simulink model "virtual_nonVirtual_CodeGeneration"  (R2024a)
settings: Solver=FixedStepDiscrete  StartTime=0.0  StopTime=10.0  FixedStep=0.5  MaxStep=1  RelTol=1
settings Model: Creator=DELL  LastModifiedBy=DELL
settings OptimizationCC: DefaultParameterBehavior=Inlined  EnhancedBackFolding=on  PassReuseOutputArgsAs=Individual arguments  ZeroExternalMemoryAtStartup=off  ZeroInternalMemoryAtStartup=off  OptimizeBlockOrder=speed  DifferentSizesBufferReuse=on  OptimizationCustomize=off  EfficientTunableParamExpr=on
settings DebuggingCC: ParameterTunabilityLossMsg=error
settings SFSimCC: MATLABDynamicMemAlloc=off
settings RTWCC: Description=Embedded Coder  SystemTargetFile=ert.tlc  TemplateMakefile=ert_default_tmf
settings CodeAppCC: ForceParamTrailComments=on  IgnoreCustomStorageClasses=off  OperatorAnnotations=on  SimulinkDataObjDesc=on  SFDataObjDesc=on  InsertBlockDesc=on
settings ERTTargetCC: TargetLangStandard=C99 (ISO)  GenerateSampleERTMain=on  InlinedParameterPlacement=NonHierarchical  ERTCustomFileTemplate=example_file_process.tlc

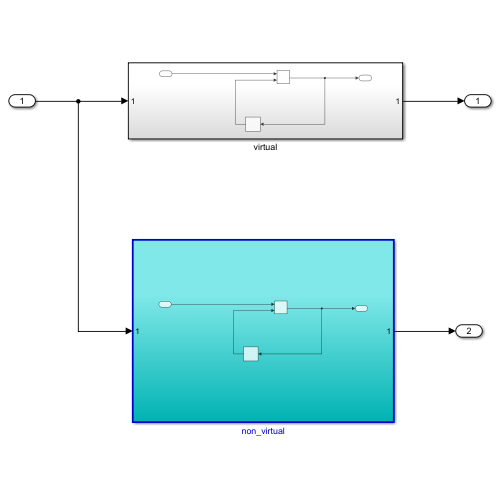
[thumbnail: Simulink's stored preview of the top-level diagram]
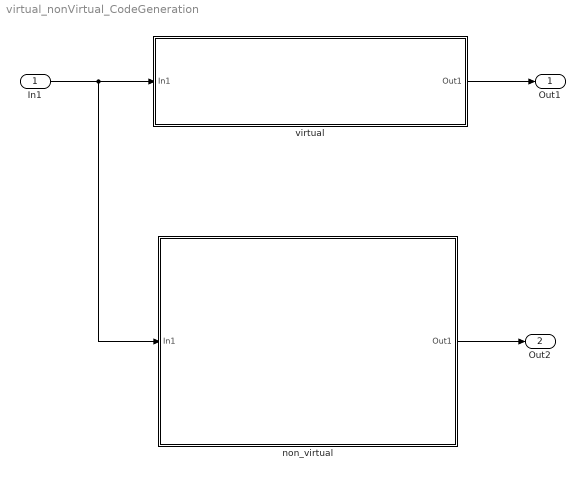
== system virtual_nonVirtual_CodeGeneration ==
  In1 : Inport
  non_virtual : Subsystem  TreatAsAtomicUnit=on  RTWFcnName=Non_V
      settings: RTWSystemCode=Nonreusable function
  virtual : Subsystem
  Out1 : Outport
  Out2 : Outport  Port=2
  wires:
  In1/1 -> non_virtual/1(In1), virtual/1(In1)
  virtual/1(Out1) -> Out1/1
  non_virtual/1(Out1) -> Out2/1

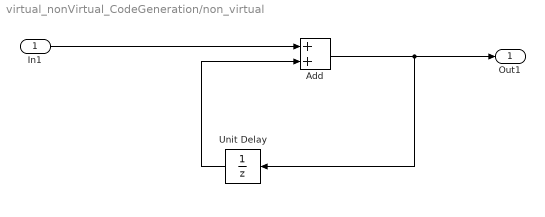
== system virtual_nonVirtual_CodeGeneration/non_virtual ==
  In1 : Inport
  Add : Sum
  Unit Delay : UnitDelay  SampleTime=-1  HasFrameUpgradeWarning=on
  Out1 : Outport
  wires:
  Unit Delay/1 -> Add/2
  In1/1 -> Add/1
  Add/1 -> Unit Delay/1, Out1/1

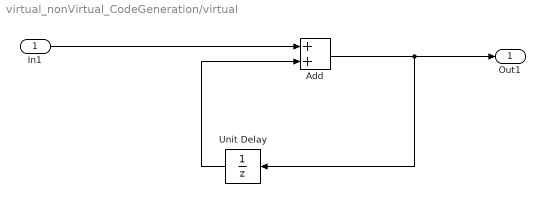
== system virtual_nonVirtual_CodeGeneration/virtual ==
  In1 : Inport
  Add : Sum
  Unit Delay : UnitDelay  SampleTime=-1  HasFrameUpgradeWarning=on
  Out1 : Outport
  wires:
  Add/1 -> Unit Delay/1, Out1/1
  Unit Delay/1 -> Add/2
  In1/1 -> Add/1
